simulink model "nCORTEx5"  (R2017b)
settings: Solver=ode4  StartTime=0.0  StopTime=inf  FixedStep=1e-3  RelTol=1e-3  EnableMultiTasking=on
libraries: xpcnilib x15, slrtlib x11
settings Model: Creator=qiwang  LastModifiedBy=Datatron
settings DataIOCC: LimitDataPoints=on  SaveFormat=StructureWithTime
settings OptimizationCC: BlockReduction=off  OptimizeBlockIOStorage=off  BufferReuse=off  GlobalBufferReuse=off  ExpressionFolding=off  LocalBlockOutputs=off  LifeSpan=inf
settings DebuggingCC: UnderspecifiedInitializationDetection=Classic  MergeDetectMultiDrivingBlocksExec=none  SolverPrmCheckMsg=warning  StateNameClashWarn=warning  SFUnexpectedBacktrackingDiag=warning  SFNoUnconditionalDefaultTransitionDiag=warning  SFExecutionAtInitializationDiag=none
settings HardwareCC: ProdBitPerPointer=32  ProdBitPerSizeT=32  ProdBitPerPtrDiffT=32  ProdLargestAtomicFloat=None  ProdWordSize=32  ProdLongLongMode=on  ProdHWDeviceType=Generic->32-bit x86 compatible
settings ModelReferenceCC: PropagateSignalLabelsOutOfModel=off
settings RTWCC: SystemTargetFile=slrt.tlc  TemplateMakefile=slrt_default_tmf  Description=Simulink Real-Time  CodeExecutionProfiling=on  RTWCompilerOptimization=on
settings CodeAppCC: StateflowObjectComments=on
settings ConfigComp: CovMetricSettings=dw  CovHtmlReporting=on  CovSaveCumulativeToWorkspaceVar=on  CovSaveSingleToWorkspaceVar=on  CovExternalEMLEnable=off

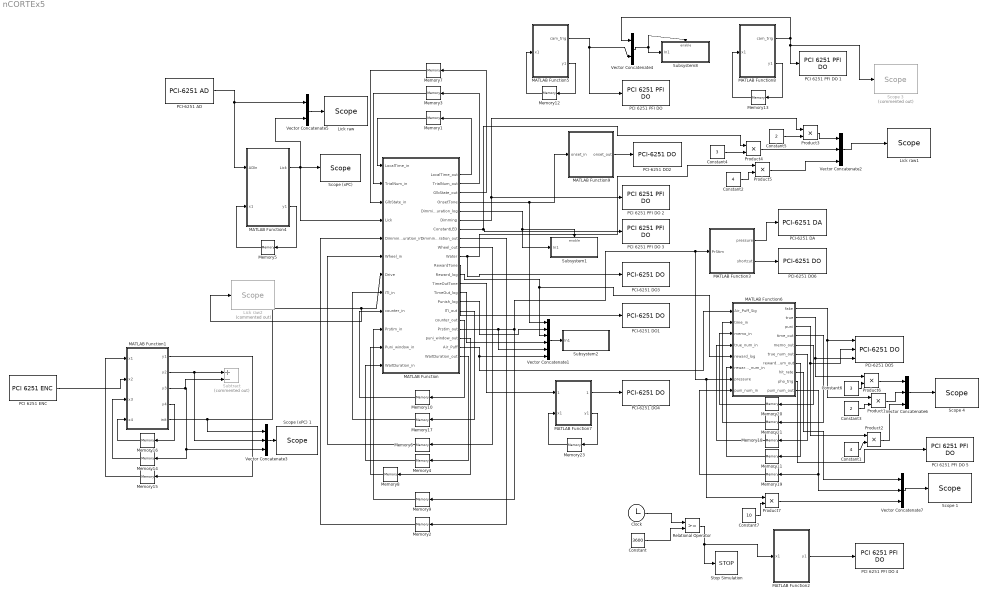
== system nCORTEx5 ==
  Clock : Clock
      settings: Decimation=1000
  Constant : Constant  Value=3600
  Constant1 : Constant  Value=4  OutDataTypeStr=double
  Constant2 : Constant  Value=4  OutDataTypeStr=double
  Constant3 : Constant  Value=2  OutDataTypeStr=double
  Constant4 : Constant  Value=3  OutDataTypeStr=double
  Constant5 : Constant  Value=2  OutDataTypeStr=double
  Constant6 : Constant  Value=3  OutDataTypeStr=double
  Constant7 : Constant  Value=10  OutDataTypeStr=double
  Lick raw : slrtlib/Displays and Logging/Scope   scopeno=1  scopetype=Target  autostart=on  viewmode=Graphical redraw  formatstr='%15.6f'  grid=on  ylimits=[-1,5]  nosamples=500  noprepostsamples=0  interleave=1  triggermode=FreeRun  triggersignal=1  trigsignalfromport=off  triggerlevel=0.0  triggerslope=Either  triggerscope=1  triggersample=0  filename=data.dat  mode=Lazy  writesize=512  autorestart=off  dynamicfilemode=off  maxwritefilesize=512*1024^2
  Lick raw1 : slrtlib/Displays and Logging/Scope   scopeno=3  scopetype=Target  autostart=on  viewmode=Graphical redraw  formatstr='%15.6f'  grid=on  ylimits=[-1,5]  nosamples=500  noprepostsamples=0  interleave=1  triggermode=FreeRun  triggersignal=1  trigsignalfromport=off  triggerlevel=0.0  triggerslope=Either  triggerscope=1  triggersample=0  filename=data.dat  mode=Lazy  writesize=512  autorestart=off  dynamicfilemode=off  maxwritefilesize=512*1024^2
  Lick raw2 : slrtlib/Displays and Logging/Scope   Commented=on  scopeno=1  scopetype=Target  autostart=on  viewmode=Graphical redraw  formatstr='%15.6f'  grid=on  ylimits=[-1,5]  nosamples=250  noprepostsamples=0  interleave=1  triggermode=FreeRun  triggersignal=1  trigsignalfromport=off  triggerlevel=0.0  triggerslope=Either  triggerscope=1  triggersample=0  filename=data.dat  mode=Lazy  writesize=512  autorestart=off  dynamicfilemode=off  maxwritefilesize=512*1024^2
  MATLAB Function : MATLAB Function  TreatAsAtomicUnit=on
  MATLAB Function1 : MATLAB Function  TreatAsAtomicUnit=on
  MATLAB Function2 : MATLAB Function  TreatAsAtomicUnit=on
  MATLAB Function3 : MATLAB Function  TreatAsAtomicUnit=on
  MATLAB Function4 : MATLAB Function  TreatAsAtomicUnit=on
  MATLAB Function5 : MATLAB Function  TreatAsAtomicUnit=on
  MATLAB Function6 : MATLAB Function  TreatAsAtomicUnit=on
  MATLAB Function7 : MATLAB Function  TreatAsAtomicUnit=on
  MATLAB Function8 : MATLAB Function  TreatAsAtomicUnit=on
  MATLAB Function9 : MATLAB Function  TreatAsAtomicUnit=on
  Memory{1..21} (21 alike) : Memory
  Memory23 : Memory  InitialCondition=1
  "PCI 6251 ENC " : xpcnilib/Incremental Encoder/PCI 6251 ENC   channel=0  countMode=Quadrature Mode x1  initCount=0  reload=off  indexPhase=A high B low  filter=None  sampleTime=0.001  slot=-1
      settings: SourceProductName=Simulink Real-Time  SourceProductBaseCode=XP
  "PCI 6251 PFI DO " : xpcnilib/Digital Output/M Series/PCI 6251 PFI DO   channel=[15]  reset=[0]  initial=[0]  sampleTime=0.001  slot=-1
      settings: SourceProductName=Simulink Real-Time  SourceProductBaseCode=XP
  PCI 6251 PFI DO 1 : xpcnilib/Digital Output/M Series/PCI 6251 PFI DO   channel=[6]  reset=[0]  initial=[0]  sampleTime=0.001  slot=-1
      settings: SourceProductName=Simulink Real-Time  SourceProductBaseCode=XP
  PCI 6251 PFI DO 2 : xpcnilib/Digital Output/M Series/PCI 6251 PFI DO   channel=[5]  reset=[0]  initial=[0]  sampleTime=0.001  slot=-1
      settings: SourceProductName=Simulink Real-Time  SourceProductBaseCode=XP
  PCI 6251 PFI DO 3 : xpcnilib/Digital Output/M Series/PCI 6251 PFI DO   channel=[4]  reset=[0]  initial=[0]  sampleTime=0.001  slot=-1
      settings: SourceProductName=Simulink Real-Time  SourceProductBaseCode=XP
  PCI 6251 PFI DO 4 : xpcnilib/Digital Output/M Series/PCI 6251 PFI DO   channel=[7]  reset=[0]  initial=[0]  sampleTime=0.001  slot=-1
      settings: SourceProductName=Simulink Real-Time  SourceProductBaseCode=XP
  PCI 6251 PFI DO 5 : xpcnilib/Digital Output/M Series/PCI 6251 PFI DO   channel=[11]  reset=[0]  initial=[0]  sampleTime=0.001  slot=-1
      settings: SourceProductName=Simulink Real-Time  SourceProductBaseCode=XP
  PCI-6251 AD : xpcnilib/A//D/M Series/PCI-6251 AD  channel=[1]  range=[10]  coupling=[0]  scantime=5e-6  sampletime=0.001  slot=-1
      settings: SourceProductName=Simulink Real-Time  SourceProductBaseCode=XP
  PCI-6251 DA : xpcnilib/D//A/M Series/PCI-6251 DA  channel=[1]  range=[10]  reset=[1]  initValue=[0]  sampletime=0.001  slot=-1
      settings: SourceProductName=Simulink Real-Time  SourceProductBaseCode=XP
  PCI-6251 DO1 : xpcnilib/Digital Output/M Series/PCI-6251 DO  channel=[1]  reset=[1]  initValue=[0]  sampletime=0.001  slot=-1
      settings: SourceProductName=Simulink Real-Time  SourceProductBaseCode=XP
  PCI-6251 DO2 : xpcnilib/Digital Output/M Series/PCI-6251 DO  channel=[2]  reset=[1]  initValue=[0]  sampletime=0.001  slot=-1
      settings: SourceProductName=Simulink Real-Time  SourceProductBaseCode=XP
  PCI-6251 DO3 : xpcnilib/Digital Output/M Series/PCI-6251 DO  channel=[4]  reset=[1]  initValue=[0]  sampletime=0.001  slot=-1
      settings: SourceProductName=Simulink Real-Time  SourceProductBaseCode=XP
  PCI-6251 DO4 : xpcnilib/Digital Output/M Series/PCI-6251 DO  channel=[3]  reset=[1]  initValue=[0]  sampletime=0.001  slot=-1
      settings: SourceProductName=Simulink Real-Time  SourceProductBaseCode=XP
  PCI-6251 DO5 : xpcnilib/Digital Output/M Series/PCI-6251 DO  channel=[8 6 5]  reset=[1]  initValue=[0]  sampletime=0.001  slot=-1
      settings: SourceProductName=Simulink Real-Time  SourceProductBaseCode=XP
  PCI-6251 DO6 : xpcnilib/Digital Output/M Series/PCI-6251 DO  channel=[7]  reset=[1]  initValue=[0]  sampletime=0.001  slot=-1
      settings: SourceProductName=Simulink Real-Time  SourceProductBaseCode=XP
  Product{1..7} (7 alike) : Product
  Relational Operator : RelationalOperator  OutDataTypeStr=boolean  RndMeth=Simplest
  "Scope (xPC) " : slrtlib/Displays and Logging/Scope   scopeno=6  scopetype=File  autostart=on  viewmode=Graphical redraw  formatstr='%15.6f'  grid=on  ylimits=[0,0]  nosamples=512  noprepostsamples=0  interleave=1  triggermode=FreeRun  triggersignal=1  trigsignalfromport=off  triggerlevel=0.0  triggerslope=Either  triggerscope=1  triggersample=0  filename=Licks.dat  mode=Lazy  writesize=512  autorestart=on  dynamicfilemode=off  maxwritefilesize=512*1024^2
  Scope (xPC) 1 : slrtlib/Displays and Logging/Scope   scopeno=7  scopetype=File  autostart=on  viewmode=Graphical redraw  formatstr='%15.6f'  grid=on  ylimits=[0,0]  nosamples=512  noprepostsamples=0  interleave=1  triggermode=FreeRun  triggersignal=1  trigsignalfromport=off  triggerlevel=0.0  triggerslope=Either  triggerscope=1  triggersample=0  filename=SelfInit.dat  mode=Lazy  writesize=512  autorestart=on  dynamicfilemode=off  maxwritefilesize=512*1024^2
  Scope 1 : slrtlib/Displays and Logging/Scope   scopeno=9  scopetype=Target  autostart=on  viewmode=Numerical  formatstr='%15.6f'  grid=on  ylimits=[-100,100]  nosamples=3  noprepostsamples=0  interleave=3  triggermode=FreeRun  triggersignal=1  trigsignalfromport=off  triggerlevel=0.0  triggerslope=Either  triggerscope=1  triggersample=0  filename=data.dat  mode=Lazy  writesize=512  autorestart=off  dynamicfilemode=off  maxwritefilesize=512*1024^2
  Scope 3 : slrtlib/Displays and Logging/Scope   Commented=on  scopeno=5  scopetype=Target  autostart=on  viewmode=Graphical redraw  formatstr='%15.6f'  grid=on  ylimits=[0,0]  nosamples=250  noprepostsamples=0  interleave=1  triggermode=FreeRun  triggersignal=1  trigsignalfromport=off  triggerlevel=0.0  triggerslope=Either  triggerscope=1  triggersample=0  filename=data.dat  mode=Lazy  writesize=512  autorestart=off  dynamicfilemode=off  maxwritefilesize=512*1024^2
  Scope 4 : slrtlib/Displays and Logging/Scope   scopeno=5  scopetype=Target  autostart=on  viewmode=Graphical redraw  formatstr='%15.6f'  grid=on  ylimits=[-1,5]  nosamples=500  noprepostsamples=0  interleave=1  triggermode=FreeRun  triggersignal=1  trigsignalfromport=off  triggerlevel=0.0  triggerslope=Either  triggerscope=1  triggersample=0  filename=data.dat  mode=Lazy  writesize=512  autorestart=off  dynamicfilemode=off  maxwritefilesize=512*1024^2
  Stop Simulation : Stop
  Subsystem1 : Subsystem
  Subsystem2 : Subsystem
  Subsystem8 : Subsystem
  Subtract : Sum  Commented=on  Inputs=+-
  Vector Concatenate1 : Concatenate  NumInputs=6
  Vector Concatenate{2..3,6..7} (4 alike) : Concatenate  NumInputs=3
  Vector Concatenate4 : Concatenate
  Vector Concatenate5 : Concatenate
  wires:
  MATLAB Function/1(LocalTime_out) -> Memory1/1
  Memory1/1 -> MATLAB Function/1(LocalTime_in)
  MATLAB Function/2(TrialNum_out) -> Memory3/1
  Memory3/1 -> MATLAB Function/2(TrialNum_in)
  MATLAB Function/3(GlbState_out) -> Memory7/1
  Memory7/1 -> MATLAB Function/3(GlbState_in)
  MATLAB Function5/2(y1) -> Memory12/1
  Memory12/1 -> MATLAB Function5/1(x1)
  MATLAB Function5/1(cam_trig) -> "PCI 6251 PFI DO "/1, Vector Concatenate4/2
  MATLAB Function4/2(y1) -> Memory5/1
  Memory5/1 -> MATLAB Function4/2(x1)
  MATLAB Function7/2(y1) -> Memory23/1
  Memory23/1 -> MATLAB Function7/2(x1)
  MATLAB Function7/1(TO_tone) -> PCI-6251 DO4/1
  MATLAB Function8/2(y1) -> Memory13/1
  Memory13/1 -> MATLAB Function8/1(x1)
  MATLAB Function8/1(cam_trig) -> PCI 6251 PFI DO 1/1, Scope 3/1, Vector Concatenate4/1
  Vector Concatenate4/1 -> Subsystem8/Enable, Subsystem8/1(In1)
  Vector Concatenate5/1 -> Lick raw/1
  MATLAB Function4/1(Lick) -> "Scope (xPC) "/1, MATLAB Function/4(Lick), Vector Concatenate5/2
  PCI-6251 AD/1 -> MATLAB Function4/1(ADIn), Vector Concatenate5/1
  "PCI 6251 ENC "/1 -> MATLAB Function1/2(x2)
  Memory14/1 -> MATLAB Function1/3(x3)
  MATLAB Function1/2(y2) -> Subtract/1, Vector Concatenate3/2
  MATLAB Function1/3(y3) -> Subtract/2, Vector Concatenate3/3, Memory14/1
  MATLAB Function1/5(init) -> Vector Concatenate3/1, Lick raw2/1, MATLAB Function/7(Drive)
  MATLAB Function1/4(y4) -> Memory16/1
  MATLAB Function1/1(y1) -> Memory15/1
  Memory15/1 -> MATLAB Function1/1(x1)
  Memory16/1 -> MATLAB Function1/4(x4)
  MATLAB Function/17(counter_out) -> Memory10/1
  MATLAB Function/9(Wheel_out) -> Memory6/1
  Memory6/1 -> MATLAB Function/6(Wheel_in)
  Memory17/1 -> MATLAB Function/8(ITI_in)
  Memory10/1 -> MATLAB Function/9(counter_in)
  MATLAB Function/8(DimmingDuration_out) -> Memory2/1
  Memory2/1 -> MATLAB Function/5(DimmingDuration_in)
  MATLAB Function/16(ITI_out) -> Memory17/1
  MATLAB Function/4(OnsetTone) -> MATLAB Function9/1(onset_in), Vector Concatenate1/1
  MATLAB Function/13(TimeOutTone) -> MATLAB Function7/1(TO_flag)
  MATLAB Function/5(DimmingDuration_log) -> Subsystem1/Enable, Subsystem1/1(In1)
  MATLAB Function/6(Dimming) -> Product3/1, PCI 6251 PFI DO 2/1
  MATLAB Function/7(ConstantLED) -> PCI 6251 PFI DO 3/1, Product4/1
  Vector Concatenate1/1 -> Subsystem2/1(In1)
  MATLAB Function/11(RewardTone) -> PCI-6251 DO1/1
  MATLAB Function/15(Punish_log) -> Vector Concatenate1/2
  MATLAB Function/14(TimeOut_log) -> Vector Concatenate1/4
  MATLAB Function/12(Reward_log) -> MATLAB Function6/5(reward_log), Vector Concatenate1/3
  Vector Concatenate2/1 -> Lick raw1/1
  Vector Concatenate3/1 -> Scope (xPC) 1/1
  Relational Operator/1 -> Stop Simulation/1, MATLAB Function2/1(x1)
  Constant/1 -> Relational Operator/2
  MATLAB Function2/1(y1) -> PCI 6251 PFI DO 4/1
  Clock/1 -> Relational Operator/1
  MATLAB Function/19(puni_window_out) -> Memory8/1
  MATLAB Function/21(WaitDuration_out) -> Memory4/1
  Memory4/1 -> MATLAB Function/12(WaitDuration_in)
  Memory8/1 -> MATLAB Function/11(Puni_window_in)
  Memory9/1 -> MATLAB Function/10(Prstim_in)
  MATLAB Function6/1(fake) -> PCI-6251 DO5/1, Product1/1
  Vector Concatenate6/1 -> Scope 4/1
  MATLAB Function6/2(true) -> PCI-6251 DO5/3, Product6/1
  MATLAB Function6/3(puni) -> PCI-6251 DO5/2, Product2/1
  Product2/1 -> Vector Concatenate6/3
  Constant1/1 -> Product2/2
  MATLAB Function6/4(time_out) -> Memory21/1
  Memory20/1 -> MATLAB Function6/3(memo_in)
  MATLAB Function/20(Air_Puff) -> Vector Concatenate1/6, MATLAB Function6/1(Air_Puff_Sig)
  Memory21/1 -> MATLAB Function6/2(time_in)
  MATLAB Function6/5(memo_out) -> Memory20/1
  Constant3/1 -> Product1/2
  Product1/1 -> Vector Concatenate6/2
  MATLAB Function3/1(pressure) -> PCI-6251 DA/1
  MATLAB Function3/2(shortcut) -> PCI-6251 DO6/1
  MATLAB Function/18(Prstim_out) -> Vector Concatenate1/5, Product7/1, MATLAB Function6/7(pressure), MATLAB Function3/1(PrStim), Memory9/1
  MATLAB Function9/1(onset_out) -> PCI-6251 DO2/1
  MATLAB Function/10(Water) -> Product5/1, PCI-6251 DO3/1
  Product3/1 -> Vector Concatenate2/1
  Product4/1 -> Vector Concatenate2/2
  Product5/1 -> Vector Concatenate2/3
  Constant2/1 -> Product5/2
  Constant4/1 -> Product4/2
  Constant5/1 -> Product3/2
  Constant6/1 -> Product6/2
  Product6/1 -> Vector Concatenate6/1
  MATLAB Function6/8(hit_rate) -> Vector Concatenate7/1
  MATLAB Function6/7(reward_num_out) -> Memory11/1
  Memory11/1 -> MATLAB Function6/6(reward_num_in)
  MATLAB Function6/6(true_num_out) -> Memory18/1
  Memory18/1 -> MATLAB Function6/4(true_num_in)
  MATLAB Function6/9(pho_trig) -> PCI 6251 PFI DO 5/1
  MATLAB Function6/10(puni_num_out) -> Vector Concatenate7/2, Memory19/1
  Vector Concatenate7/1 -> Scope 1/1
  Memory19/1 -> MATLAB Function6/8(puni_num_in)
  Constant7/1 -> Product7/2
  Product7/1 -> Vector Concatenate7/3

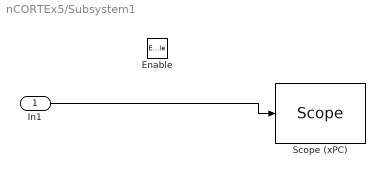
== system nCORTEx5/Subsystem1 ==
  In1 : Inport
  Enable : EnablePort
  "Scope (xPC) " : slrtlib/Displays and Logging/Scope   scopeno=4  scopetype=File  autostart=on  viewmode=Graphical redraw  formatstr='%15.6f'  grid=on  ylimits=[0,0]  nosamples=512  noprepostsamples=0  interleave=1  triggermode=FreeRun  triggersignal=1  trigsignalfromport=off  triggerlevel=0.0  triggerslope=Either  triggerscope=1  triggersample=0  filename=DimTime.dat  mode=Lazy  writesize=512  autorestart=on  dynamicfilemode=off  maxwritefilesize=512*1024^2
  wires:
  In1/1 -> "Scope (xPC) "/1

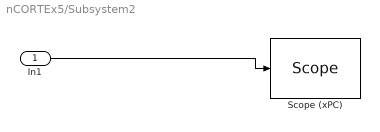
== system nCORTEx5/Subsystem2 ==
  In1 : Inport
  "Scope (xPC) " : slrtlib/Displays and Logging/Scope   scopeno=2  scopetype=File  autostart=on  viewmode=Graphical redraw  formatstr='%15.6f'  grid=on  ylimits=[0,0]  nosamples=512  noprepostsamples=0  interleave=1  triggermode=FreeRun  triggersignal=1  trigsignalfromport=off  triggerlevel=0.0  triggerslope=Either  triggerscope=1  triggersample=0  filename=Tones.dat  mode=Lazy  writesize=512  autorestart=on  dynamicfilemode=off  maxwritefilesize=512*1024^2
  wires:
  In1/1 -> "Scope (xPC) "/1

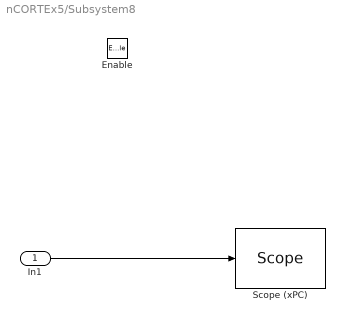
== system nCORTEx5/Subsystem8 ==
  In1 : Inport
  Enable : EnablePort
  "Scope (xPC) " : slrtlib/Displays and Logging/Scope   scopeno=13  scopetype=File  autostart=on  viewmode=Graphical redraw  formatstr='%15.6f'  grid=on  ylimits=[0,0]  nosamples=512  noprepostsamples=0  interleave=1  triggermode=FreeRun  triggersignal=1  trigsignalfromport=off  triggerlevel=0.0  triggerslope=Either  triggerscope=1  triggersample=0  filename=CmraTrig.dat  mode=Lazy  writesize=512  autorestart=on  dynamicfilemode=off  maxwritefilesize=512*1024^2
  wires:
  In1/1 -> "Scope (xPC) "/1

== matlab function nCORTEx5/MATLAB Function1 ==
  data: x1 input; y1 output; y2 output; y3 output; x2 input; x3 input; x4 input; y4 output; init output
function [y1, y2, y3, y4, init] = WheelDriving(x1, x2, x3, x4)
% detect wheel locomotion
% y1: clk
% y2: RT-readout
% y3: history-readout
% y4: flag
if x1 == 0
    y1 = x1+1;
    % if trig == 0
    y2 = 0;
    y3 = 0;
    y4 = 1;
    init = 0;
else
    % else
    y4 = x4;
    y2 = x2;
    if y4 == 1
        y3 = x2;
        y4 = 0;
        init = 0;
        y1 = x1+1;
    else
        y3 = x3;
        diff = y2-y3;
        if diff > 10
            init = 1;
            y4 = 1;
            y1 = 0;
        elseif diff < -50
            init = -1;
            y4 = 1;
            y1 = 0;
        else
            init = 0;
            y4 = 0;
            y1 = x1+1;
        end
    end
end

== matlab function nCORTEx5/MATLAB Function ==
  data: LocalTime_in input; TrialNum_in input; GlbState_in input; LocalTime_out output; TrialNum_out output; GlbState_out output; OnsetTone output; DimmingDuration_log output; Dimming output; ConstantLED output; DimmingDuration_out output; Wheel_out output; Lick input; DimmingDuration_in input; Wheel_in input; Drive input; Water output; RewardTone output; Reward_log output; ITI_in input; TimeOutTone output; TimeOut_log output; Punish_log output; ITI_out output; counter_in input; counter_out output; Prstim_in input; Puni_window_in input; Prstim_out output; puni_window_out output; Air_Puff output; WaitDuration_in input; WaitDuration_out output
function [LocalTime_out, TrialNum_out, GlbState_out, OnsetTone, DimmingDuration_log, Dimming, ConstantLED, DimmingDuration_out, Wheel_out, Water, RewardTone, Reward_log, TimeOutTone, TimeOut_log, Punish_log, ITI_out, counter_out, Prstim_out, puni_window_out, Air_Puff, WaitDuration_out] = Main_Control(LocalTime_in, TrialNum_in, GlbState_in, Lick, DimmingDuration_in, Wheel_in, Drive, ITI_in, counter_in, Prstim_in,Puni_window_in, WaitDuration_in)
%%Andy-2021-11-28
%xPC target for head-fixed detection paradigm
%y1->x1: inernal counter
%y2->GlbState: state index
%y3->WaitDuration: internal memory for trail duration

%coder.extrinsic('rng');
coder.cinclude('"time.h"');
sd = 0;
sd = coder.ceval('time',[]);
rng(sd,'twister');

switch (GlbState_in)
    case {0} % Start LED dimming at the beginning of each trial
        %% 
        counter_out=counter_in+1;
        OnsetTone = 0; % trigger the Arduino board to generate Trial Onset Tone, OnsetTone =-1 means a trial (passive activated) start, and OnsetTone =2 means a new SSD part start (self activated trial)
        Dimming = 0;
        ConstantLED = 0;
        GlbState_out = 6; % go to state 1
        DimmingDuration_out = 0;  %% %LED blink duration: 4-6 s
        DimmingDuration_log = DimmingDuration_out;
        LocalTime_out = 0;
        ITI_out = ITI_in;
        TrialNum_out = TrialNum_in + 1;
        Water = 0;
        RewardTone = 0;
        Wheel_out = 0;
        TimeOutTone = 0;
        Reward_log = 0;
        TimeOut_log = 0;
        Punish_log = 0;
        Prstim_out = Prstim_in;
        puni_window_out = 0;
        Air_Puff = 0; % Air_Puff = 0 means no puff at all; Air_Puff = 1 means a stimulation coupled with a distractor; Air_Puff = -1 means a distractor puff only,  
        %Air_Puff = -2 means a punishment puff; and Air_Puff = -3 means a
        %0psi stimulation coupled with a distractor
        WaitDuration_out= WaitDuration_in;
case {4} 
    %% no-lick period: 2000ms (if animal licks, start over)
        counter_out=counter_in+1;
        Prstim_out = Prstim_in;
        Punish_log = 0;
        sd = coder.ceval('time',[]);
        rng(sd+counter_in,'twister');
        if LocalTime_in < 2000
            GlbState_out = 4; %self loop
            if Lick ~= 0  % animal licked, add a random delay
                tmp = rand(1);
                Punish_log = 1; %small punishment due to impulsive lick is logged as 1 and harsh punishment due to distracted lick is logged as 2,
                LocalTime_out = -1*(1000+tmp*4000); %rest and a punishment of waiting 1-4s;
            else
                LocalTime_out = LocalTime_in + 1;
            end
        else
            LocalTime_out = 0;
            GlbState_out = 8;%Go to stimulation delivery               
        end
        
        TrialNum_out = TrialNum_in;
        OnsetTone = 0;
        Dimming = 0;
        ConstantLED = 0;
        DimmingDuration_out = 0;
        DimmingDuration_log = DimmingDuration_out;
        ITI_out = ITI_in;
        RewardTone = 0;
        Wheel_out = 0;
        TimeOutTone = 0;
        Reward_log = 0;
        TimeOut_log = 0;
       
        Water = 0;
        WaitDuration_out = WaitDuration_in;
        
        Air_Puff = 0;%No air-puff in most cases
        if Puni_window_in > 0 
            if Lick ~= 0
                GlbState_out = 11; % go to harsh punishment
                Punish_log = 2; % !!! small punishment due to impulsive lick is logged as 1 and harsh punishment due to distracted lick is logged as 2, timeout due to turning wheel right is 3
                LocalTime_out = 0;
                puni_window_out = 0;
            else 
                puni_window_out=Puni_window_in-1;
            end
        else
            puni_window_out=Puni_window_in;
        end
        sd = coder.ceval('time',[]);
        rng(sd+counter_in,'twister');
        tmp = rand(1);
        if tmp<0.00015 %Low possibility determined every time point to trigger a random distractor
            Air_Puff=-1; % distractor puff
            %reset punishment window
            puni_window_out=1000;
        end
        
    case {5} % ITI
        %% 
        counter_out=counter_in+1;
        ITI_out = ITI_in;
        LocalTime_out = LocalTime_in+1;
        if LocalTime_out < ITI_out
            GlbState_out = 5;
        else
            GlbState_out = 0;
            LocalTime_out = 0;
        end
        
        Dimming = 0;
        DimmingDuration_out = DimmingDuration_in;
        ConstantLED = 0;
        DimmingDuration_log = 0;
        TrialNum_out = TrialNum_in;
        OnsetTone = 0;
        Water = 0;
        RewardTone = 0;
        Wheel_out = 0;
%         Wheel_trig = 0;
        TimeOutTone = 0;
        Reward_log = 0;
        TimeOut_log = 0;
        Punish_log = 0;
        Prstim_out = Prstim_in;
        puni_window_out = 0;
        Air_Puff = 0;
        WaitDuration_out= WaitDuration_in;

case {6} 
    %% Puff Detection part start:
    % A 1ms state with no Random Distractor. This state turns off lights, 
    % decide puff strenth and length of the random waiit after the start
        counter_out=counter_in+1;
        OnsetTone = 1; % trigger the Arduino board to generate Trial Onset Tone
        GlbState_out = 7; % go to state 7, the wait period with distractor
        sd = coder.ceval('time',[]);
        rng(sd+counter_in,'twister');
        tmp = rand(1);
        WaitDuration_out = (8000+(tmp*8000));  %% %Delay before stim start: 8-16 s
        LocalTime_out = 0;
        puni_window_out = 0;
        Dimming = 0;
        
        TrialNum_out = TrialNum_in;
        %PrStim = 0; %later changed to PrStim = Stim_out; 
        Water = 0;
        RewardTone = 0;
        TimeOutTone = 0;
        Air_Puff = 0;
        ConstantLED = 0;
        DimmingDuration_out = DimmingDuration_in;
        DimmingDuration_log = 0;
        Wheel_out = 0;
        Reward_log = 0;
        TimeOut_log = 0;
        Punish_log = 0;
        ITI_out = ITI_in;
        
        % determine which stimulus pressure to use among 1,2,5 and 10 Psi
%         sd = coder.ceval('time',[]);
%         rng(sd,'twister');
        tmp = rand(1);
        % !!! what voltage signal should be given to the pressure valve?
        % 0-10v = 0-100psi
        if tmp < 1/7 %true 0psi, true stimulation wont fire
            Prstim_out = 0;
        elseif tmp < 2/7 %0.5Psi
            Prstim_out = 0.05;
        elseif tmp < 3/7 %1Psi
            Prstim_out = 0.1;
        elseif tmp < 4/7 %2Psi
            Prstim_out = 0.2;
        elseif tmp < 5/7 %5Psi
            Prstim_out = 0.5;            
        elseif tmp < 6/7%10Psi
            Prstim_out = 1.0;
        else %20Psi
            Prstim_out = 2.0;
        end       

	case {7} 
        %% Distractor window:
        %lights off, random distractors emerge with punishment window
        %that will punish the mouse if it licks in this window
        counter_out=counter_in+1;
        if LocalTime_in < WaitDuration_in
            GlbState_out = 7; % self loop
            LocalTime_out = LocalTime_in + 1;            
        else
            LocalTime_out = 0;
            GlbState_out = 4; % Go to No lick period        
        end
        
        Prstim_out = Prstim_in; %to control pressure valve
        TrialNum_out = TrialNum_in;
        OnsetTone = 0;
        RewardTone = 0;
        TimeOutTone = 0;
        Water = 0;
        Dimming = 0;
        ConstantLED = 0;
        DimmingDuration_out = DimmingDuration_in;
        DimmingDuration_log = 0;
        Wheel_out = 0;
        Reward_log = 0;
        TimeOut_log = 0;
        Punish_log = 0;
        ITI_out = ITI_in;
        
        Air_Puff = 0; %No air-puff in most cases
        if Puni_window_in > 0 
            if Lick ~= 0
                GlbState_out = 11; % go to harsh punishment
                Punish_log = 2; % !!! small punishment due to impulsive lick is logged as 1 and harsh punishment due to distracted lick is logged as 2, timeout due to turning wheel right is 3
                LocalTime_out = 0;
                puni_window_out = 0;
            else 
                puni_window_out=Puni_window_in-1;
            end
        else
            puni_window_out=Puni_window_in;
        end
        sd = coder.ceval('time',[]);
        rng(sd+counter_in,'twister');
        tmp = rand(1);
        if tmp<0.00015 %Low possibility determined every time point to trigger a random distractor
            Air_Puff=-1; % distractor puff
            %reset punishment window
            puni_window_out=800;
        end
        WaitDuration_out = WaitDuration_in;
        
    case {8} 
        %% Stimulus delivery
        counter_out=counter_in+1;
        Prstim_out = Prstim_in;
        if LocalTime_in < 1
            LocalTime_out = 0;
            GlbState_out = 9; % Go to windows of opportunity
            Air_Puff = 1; %deliver true stimuli
            % !!! do we still need to use distractor as a true 0? still
            % use, but not as true 0, but always coubled with the
            % stimulation
            % !!! use shortcut strategy? yes
            if Prstim_out == 0
                Air_Puff = -3;
            end
        else
            Air_Puff = 0;
            LocalTime_out = 0;
            GlbState_out = 8; %self loop to reset LocalTime_out in case weird bug cause skipped stimulation
        end
                
        TrialNum_out = TrialNum_in;
        OnsetTone = 0;
        RewardTone = 0;
        TimeOutTone = 0;
        Water = 0;
        WaitDuration_out= WaitDuration_in;
        puni_window_out=0;
        Dimming = 0;
        ConstantLED = 0;
        DimmingDuration_out = DimmingDuration_in;
        DimmingDuration_log = 0;
        Wheel_out = 0;
        Reward_log = 0;
        TimeOut_log = 0;
        Punish_log = 0;
        ITI_out = ITI_in;

        
    case {9} 
        %% window of opportunity: 800ms
        % when the behavior/ response of the animal is evaluated and then
        % direct to different consequences on the mice including: big
        % reward, or nothing at all
        counter_out=counter_in+1;
        LocalTime_out = LocalTime_in+1;
        ITI_out = ITI_in;
        WaitDuration_out= WaitDuration_in;
        DimmingDuration_out = DimmingDuration_in;
        DimmingDuration_log = 0;
        if LocalTime_in < 800
            if Lick ~= 0
                if Prstim_in >0            
                    GlbState_out = 10; % a big reward associate with 40 psi puff
                    LocalTime_out = 0;
                    Reward_log = 2; % !!! small reward logged as 1;  big reward triggered logged as 2;  big reward dilivered after delay is logged as 3
                else
                    GlbState_out = 5; % nothing happens and go back to ITI when there is no puff
                    LocalTime_out = 0;
                    Reward_log = 0;
                end
            else
                GlbState_out = 9; %self loop: continue window of opportunity
                Reward_log = 0;
            end
        else
            GlbState_out = 5; %No response until ends of window of opportunity: could be either miss or correct reject, go to ITI
            sd = coder.ceval('time',[]);
            rng(sd+counter_in,'twister');
            tmp = rand(1);
            ITI_out = 5000+tmp*2000;
            LocalTime_out = 0;
            Reward_log = 0;
        end

        TrialNum_out = TrialNum_in;
        OnsetTone = 0;
        RewardTone = 0;
        TimeOutTone = 0;
        Water = 0;
        Prstim_out = Prstim_in;
        Air_Puff = 0;
        puni_window_out=0;
        Dimming = 0;
        ConstantLED = 0;
        Wheel_out = 0;
        TimeOut_log = 0;
        Punish_log = 0;

        
case {10} 
    %% Big reward:
    % Water pump for reward
        counter_out=counter_in+1;
        LocalTime_out = LocalTime_in + 1;
        ITI_out = ITI_in;
        if LocalTime_out < 200 % !!! here you can adjust reward for correct responding to air puff
            Water = 1;
            GlbState_out = 10;% self loop
            RewardTone = 1; % trigger Arduino board to generate reward tone
        else
            GlbState_out = 5; %the feast ends, go back to ITI
            sd = coder.ceval('time',[]);
            rng(sd+counter_in,'twister');
            tmp = rand(1);
            ITI_out = 5000+tmp*5000;
            Water = 0;
            LocalTime_out = 0;
            RewardTone = 0;
        end
        
        TrialNum_out = TrialNum_in;
        OnsetTone = 0;
        TimeOutTone = 0;
        Prstim_out = Prstim_in;
        WaitDuration_out= WaitDuration_in;
        Air_Puff = 0;
        puni_window_out=0;
        Dimming = 0;
        ConstantLED = 0;
        DimmingDuration_out = DimmingDuration_in;
        DimmingDuration_log = 0;
        Wheel_out = 0;
        Reward_log = 0;
        TimeOut_log = 0;
        Punish_log = 0;
        
        
case {11} 
    %% Harsh Punishment:
    % Give the mouse a harsh punishment if it response to the distractor:
    % including a punishing air puff, 20ms timeout tone and 15s constant led light
        counter_out=counter_in+1;
        LocalTime_out = LocalTime_in + 1;
        ITI_out = ITI_in;
        if LocalTime_out < 2 % 1ms punish airpuff signal
            Air_Puff = -2;
        else
            Air_Puff = 0;
        end
        if LocalTime_out < 1000 % 1s time out tone
            TimeOutTone = 1;
            ConstantLED = 0;
            GlbState_out = 11; %self loop
        elseif LocalTime_out < 15000 %15s timeout period+ LED
            TimeOutTone = 0;
            ConstantLED = 0;
            GlbState_out = 11; %self loop
        else
            GlbState_out = 5; % back to start
            sd = coder.ceval('time',[]);
            rng(sd+counter_in,'twister');
            tmp = rand(1);
            ITI_out = 12000+tmp*18000;
            LocalTime_out = 0;
            TimeOutTone = 0;  
            ConstantLED = 0;
        end
        TrialNum_out = TrialNum_in;
        OnsetTone = 0; 
        RewardTone = 0;
        Water = 0;
        Prstim_out = Prstim_in;
        WaitDuration_out= WaitDuration_in;
        puni_window_out=0;
        Dimming = 0;
        DimmingDuration_out = DimmingDuration_in;
        DimmingDuration_log = 0;
        Wheel_out = 0;
        Reward_log = 0;
        TimeOut_log = 0;
        Punish_log = 0;

    otherwise
        counter_out=counter_in+1;
        LocalTime_out = 0;
        GlbState_out = 0;
        Dimming = 0;
        ConstantLED = 0;
        DimmingDuration_out = DimmingDuration_in;
        DimmingDuration_log = 0;
        TrialNum_out = TrialNum_in;
        OnsetTone = 0;
        RewardTone = 0;
        Water = 0;
        Wheel_out = 0;
%         Wheel_trig = 0;
        TimeOutTone = 0;
        Reward_log = 0;
        TimeOut_log = 0;
        Punish_log = 0;
        ITI_out = ITI_in;
        Prstim_out = Prstim_in;
        puni_window_out = 0;
        Air_Puff = 0;
        WaitDuration_out= WaitDuration_in;
%         
 end

== matlab function nCORTEx5/MATLAB Function2 ==
  data: x1 input; y1 output
function y1   = photometry_trigger(x1)
%y1: clk

if x1==1
    y1=0;
else 
    y1=1;
end

== matlab function nCORTEx5/MATLAB Function3 ==
  data: PrStim input; pressure output; shortcut output
function [pressure, shortcut]  = Pressure_control(PrStim)
% !!! use shortcut strategy? yes
pressure=PrStim;
if PrStim==0
    shortcut=0;
else
    shortcut=0;
end

== matlab function nCORTEx5/MATLAB Function4 ==
  data: ADIn input; Lick output; y1 output; x1 input
function [Lick, y1] = LickDetector(ADIn, x1)
%#codegen
%y1 is internal lick counter
%y2 is time counter
%ADIn = abs(ADIn);


if ADIn >= 0.2
    y1 = x1+1; 
    if x1 > 5  %lick high > 5 ms
        Lick = 1;
    else
        Lick = 0;
    end
else
    Lick = 0;
    y1 = 0;
end

== matlab function nCORTEx5/MATLAB Function5 ==
  data: cam_trig output; x1 input; y1 output
function [cam_trig, y1]  = PupilCam(x1)
%y1: clk
% will keep sending 10 Hz pulses with 5ms high 95ms low

y1 = x1+1;
if y1 <= 10 % pulse duration = 10 ms
    cam_trig = 1;
elseif y1 < 100  % camera triggered at 10 Hz (every 100 ms)
    cam_trig = 0;
else
    y1=0;    
    cam_trig=0;
end

== matlab function nCORTEx5/MATLAB Function6 ==
  data: Air_Puff_Sig input; fake output; true output; time_in input; puni output; memo_in input; time_out output; memo_out output; true_num_in input; reward_log input; reward_num_in input; true_num_out output; reward_num_out output; hit_rate output; pressure input; pho_trig output; puni_num_in input; puni_num_out output
function [fake, true, puni ,time_out, memo_out,true_num_out, reward_num_out, hit_rate, pho_trig, puni_num_out]  = Air_Puff(Air_Puff_Sig, time_in, memo_in,true_num_in, reward_log, reward_num_in, pressure,puni_num_in)
% !!! do we still need to use distractor as a true 0? still
% use, but not as true 0, but always coubled with the
% stimulation
if Air_Puff_Sig ~= 0
    memo_out=Air_Puff_Sig;
    time_out=0;
    fake=0;
    true=0;
    puni=0;
else
    time_out=time_in+1;
    if time_out < 13
        memo_out=memo_in;
        if memo_out == 1
            fake = 1;
            true = 1;
            puni = 0;
        elseif memo_out == -1
            true = 0;
            fake = 1;
            puni = 0;
        elseif memo_out == -2
            true = 0;
            fake = 0;
            puni = 1;
        elseif memo_out == -3
            true = 1;
            fake = 1;
            puni = 0;
        else
            fake = 0;
            true = 0;
            puni = 0;
        end
    else
        fake=0;
        true=0;
        puni=0;
        memo_out=0;
    end
end

if Air_Puff_Sig == 1
    true_num_out = true_num_in +1;
else
    true_num_out = true_num_in;
end

if reward_log ~= 0
    reward_num_out = reward_num_in +1;
else
    reward_num_out = reward_num_in;
end

if reward_num_out == 0
    hit_rate = 0;
else
    hit_rate = reward_num_out/true_num_out*100;
end

if true*pressure > 0
    pho_trig = 1;
else
    pho_trig = 0;
end

if Air_Puff_Sig == -2
    puni_num_out = puni_num_in +1;
else
    puni_num_out = puni_num_in;
end

== matlab function nCORTEx5/MATLAB Function7 ==
  data: TO_flag input; TO_tone output; x1 input; y1 output
function [TO_tone,y1]  = time_out(TO_flag,x1)

if TO_flag == 0
    y1 = 0;
    TO_tone = 0;
else
    y1 = x1 + 1;
    if rem(x1,200) == 0
        TO_tone = 1;
    else
        TO_tone = 0;
    end
end

== matlab function nCORTEx5/MATLAB Function8 ==
  data: cam_trig output; x1 input; y1 output
function [cam_trig, y1]  = WhiskingCam(x1)
%y1: clk


y1 = x1+1;
if y1 <= 5 % pulse duration = 5 ms
    cam_trig = 1;
elseif y1 < 20  % camera triggered at 50 Hz (every 20 ms)
    cam_trig = 0;
else
    y1=0;    
    cam_trig=0;
end

== matlab function nCORTEx5/MATLAB Function9 ==
  data: onset_in input; onset_out output
function onset_out   = binary_onset_tone(onset_in)

if onset_in > 0
    onset_out = 1;
else
    onset_out = 0;
end

end
